simulink model "Report_13_state_feedback_only"  (R2022a)
settings: Solver=FixedStepAuto  StartTime=0.0  StopTime=10  FixedStep=1e-3  RelTol=1e-3
settings Model: Creator=takahiro  LastModifiedBy=takahiro

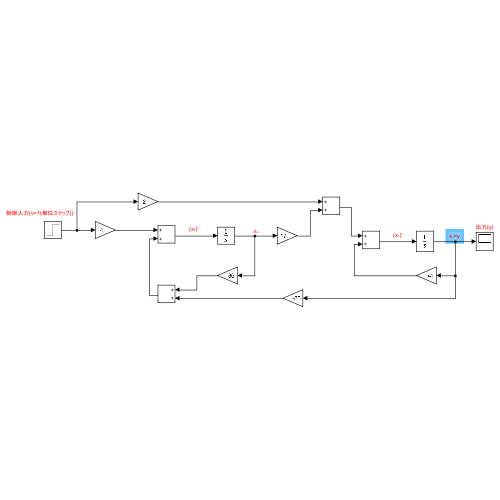
[thumbnail: Simulink's stored preview of the top-level diagram]
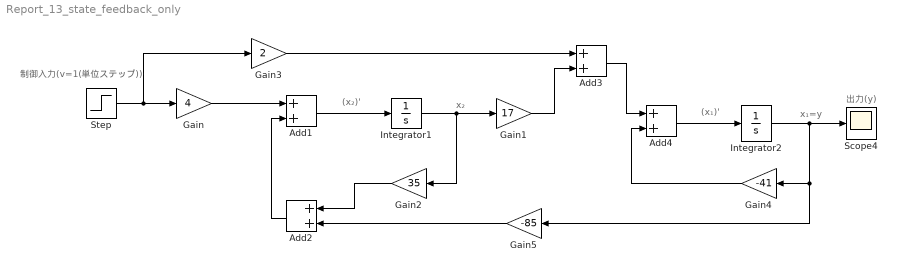
== system Report_13_state_feedback_only ==
  note: 制御入力(v=1(単位ステップ))
  note: x₁=y
  note: 出力(y)
  note: x₂
  note: (x₁)'
  note: (x₂)'
  Add{1..4} (4 alike) : Sum
  Gain : Gain  Gain=4
  Gain1 : Gain  Gain=17
  Gain2 : Gain  Gain=35
  Gain3 : Gain  Gain=2
  Gain4 : Gain  Gain=-41
  Gain5 : Gain  Gain=-85
  Integrator1 : Integrator
  Integrator2 : Integrator
  Scope4 : Scope
  Step : Step  Time=10  Before=1  SampleTime=0
  wires:
  Gain/1 -> Add1/1
  Add1/1 -> Integrator1/1
  Integrator1/1 -> Gain2/1, Gain1/1
  Gain2/1 -> Add2/1
  Add2/1 -> Add1/2
  Gain1/1 -> Add3/2
  Gain3/1 -> Add3/1
  Add3/1 -> Add4/1
  Add4/1 -> Integrator2/1
  Gain4/1 -> Add4/2
  Integrator2/1 -> Gain5/1, Gain4/1, Scope4/1
  Gain5/1 -> Add2/2
  Step/1 -> Gain3/1, Gain/1
